simulink model "mdl_r23a"  (R2023a)
settings: Solver=ode1  StartTime=0.0  StopTime=inf  FixedStep=0.1  RelTol=1e-3  EnableMultiTasking=on
values from neighbouring files (symbols this model uses):
  A = 1    [init.m]
  Cn = 30    [init.m]
  Cw = 1.1    [init.m]
  fr = 0.02    [init.m]
  g = 9.81    [init.m]
  i1 = 74/9    (= 8.22222222222)    [init.m]
  i2 = 58/10    (= 5.8)    [init.m]
  Kp = 4000    [init.m]
  m = 455    [init.m]
  m_achse_mitte = Jachse_mitte * i2*i2 / (rR*rR)    (= 1.70347629346)    [init.m]
  m_achse_unten = Jachse_unten / (rR*rR)    (= 0.877732533291)    [init.m]
  m_motor = Jmotor * i1*i1*i2*i2 / (rR*rR)    (= 38.3878032221)    [init.m]
  m_raeder = 4 * Jrad / (rR*rR)    (= 13.5035774353)    [init.m]
  rho = 1.2    [init.m]
  rR = 0.2434    [init.m]
  stop_distance = 10.6182    [init.m]
  Tn = 200    [init.m]
  Un = 48    [init.m]
undefined symbols (not defined in the file or in its folder): f_reibwert, gradient_distance_lookup, gradient_lookup, M_Motor
settings Model: Creator=roustiam  LastModifiedBy=Nico Hörter
settings SolverCC: AlgebraicLoopSolver=TrustRegion
settings DataIOCC: LimitDataPoints=on  SaveFormat=Array  SignalLoggingSaveFormat=ModelDataLogs  ReturnWorkspaceOutputs=off  SignalLoggingName=sigsOut
settings OptimizationCC: BlockReduction=off  BooleanDataType=off  ExpressionDepthLimit=2147483647  InitFltsAndDblsToZero=on  LifeSpan=inf
settings DebuggingCC: SaveWithParameterizedLinksMsg=none  UnderspecifiedInitializationDetection=Classic  MergeDetectMultiDrivingBlocksExec=none  SignalResolutionControl=TryResolveAllWithWarning  MultiTaskDSMMsg=warning  MultiTaskCondExecSysMsg=none  FcnCallInpInsideContextMsg=warning  UnconnectedInputMsg=warning  UnconnectedOutputMsg=warning  UnconnectedLineMsg=warning  StateNameClashWarn=warning  SFUnexpectedBacktrackingDiag=warning  SFNoUnconditionalDefaultTransitionDiag=warning  ArithmeticOperatorsInVariantConditions=warning
settings HardwareCC: ProdBitPerPointer=32  ProdBitPerSizeT=32  ProdBitPerPtrDiffT=32  ProdLargestAtomicFloat=None  ProdIntDivRoundTo=Undefined  ProdEndianess=Unspecified  ProdWordSize=32  ProdHWDeviceType=32-bit Generic  TargetUnknown=on
settings ModelReferenceCC: EnableRefExpFcnMdlSchedulingChecks=on  PropagateSignalLabelsOutOfModel=off
settings SFSimCC: SimUseLocalCustomCode=off  CustomCodeUndefinedFunction=UseInterfaceOnly
settings RTWCC: RTWUseLocalCustomCode=off
settings CodeAppCC: StateflowObjectComments=on
settings GRTTargetCC: TargetFcnLib=ansi_tfl_tmw.mat  TargetLangStandard=C89/C90 (ANSI)  CombineOutputUpdateFcns=off  GRTInterface=on
settings ConfigComp: CovMetricSettings=dw  CovSaveCumulativeToWorkspaceVar=on  CovSaveSingleToWorkspaceVar=on  CovExternalEMLEnable=off

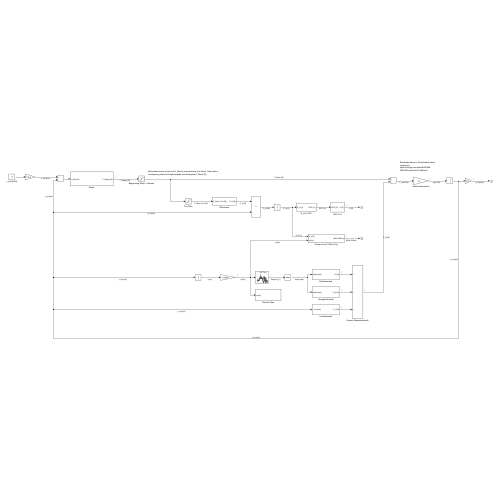
[thumbnail: Simulink's stored preview of the top-level diagram]
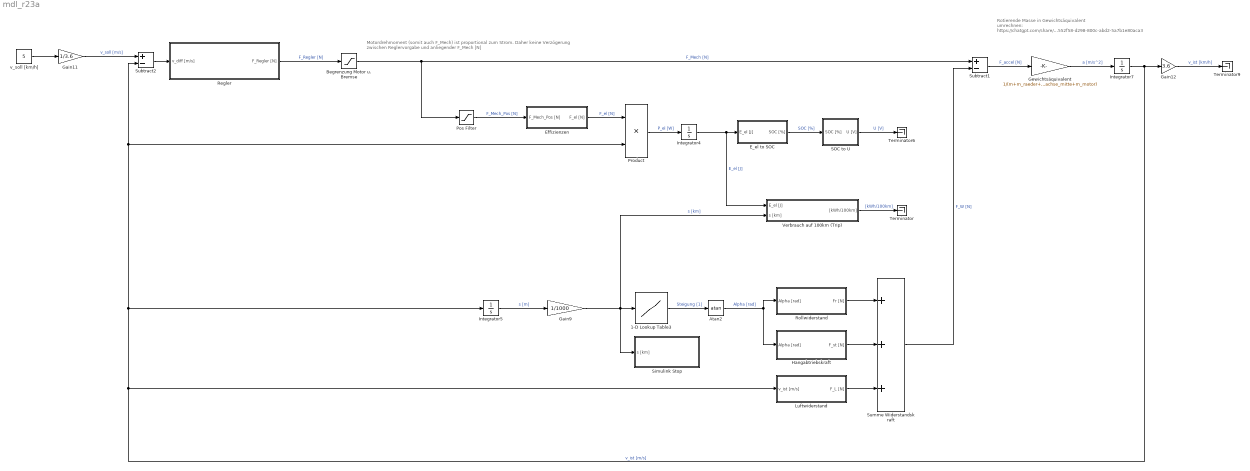
== system mdl_r23a ==
  note: Motordrehmoment (somit auch F_Mech) ist proportional zum Strom. Daher keine Verzögerung zwischen Reglervorgabe und anliegender F_Mech [N]
  note: Rotierende Masse in Gewichtsäquivalent umrechnen:
      | https://chatgpt.com/share/68552f58-d298-800c-abd2-5a7b1e80aca3
  1-D Lookup Table3 : Lookup_n-D  NumberOfTableDimensions=1  BreakpointsForDimension1=gradient_distance_lookup  Table=gradient_lookup  ExtrapMethod=Clip  InternalRulePriority=Speed  RndMeth=Simplest
  Atan2 : Trigonometry  Operator=atan
  Begrenzung Motor u. Bremse : Saturate  UpperLimit=M_Motor*i1*i2/rR  LowerLimit=-f_reibwert*m*g
  E_el to SOC : Subsystem
  Effizienzen : Subsystem
  Gain11 : Gain  Gain=1/3.6
  Gain12 : Gain  Gain=3.6
  Gain9 : Gain  Gain=1/1000
  Gewichtsäquivalent : Gain  Gain=1/(m+m_raeder+m_achse_unten+m_achse_mitte+m_motor)
  Hangabtriebskraft : Subsystem
  Integrator4 : Integrator
  Integrator5 : Integrator
  Integrator7 : Integrator
  Luftwiderstand : Subsystem
  Pos Filter : Saturate  UpperLimit=inf  LowerLimit=0
  Product : Product
  Regler : Subsystem
  Rollwiderstand : Subsystem
  SOC to U : Subsystem
  Simulink Stop : Subsystem
  Subtract1 : Sum  Inputs=+-
  Subtract2 : Sum  Inputs=+-
  Summe Widerstandskraft : Sum  Inputs=+++
  Terminator : Terminator
  Terminator6 : Terminator
  Terminator9 : Terminator
  Verbrauch auf 100km (Trip) : Subsystem
  v_soll [km/h] : Constant  Value=5
  wires:
  Atan2/1 -> Rollwiderstand/1(Alpha [rad]), Hangabtriebskraft/1(Alpha [rad])  "Alpha [rad]"
  1-D Lookup Table3/1 -> Atan2/1  "Steigung [1]"
  Gain9/1 -> Verbrauch auf 100km (Trip)/2(s [km]), Simulink Stop/1(s [km]), 1-D Lookup Table3/1  "s [km]"
  Integrator5/1 -> Gain9/1  "s [m]"
  Rollwiderstand/1(Fr [N]) -> Summe Widerstandskraft/1
  Hangabtriebskraft/1(F_st [N]) -> Summe Widerstandskraft/2
  Luftwiderstand/1(F_L [N]) -> Summe Widerstandskraft/3
  Gewichtsäquivalent/1 -> Integrator7/1  "a [m/s^2]"
  Integrator7/1 -> Product/2, Subtract2/2, Integrator5/1, Luftwiderstand/1(v_ist [m/s]), Gain12/1  "v_ist [m/s]"
  Summe Widerstandskraft/1 -> Subtract1/2  "F_W [N]"
  Regler/1(F_Regler [N]) -> Begrenzung Motor u. Bremse/1  "F_Regler [N]"
  Subtract1/1 -> Gewichtsäquivalent/1  "F_accel [N]"
  v_soll [km/h]/1 -> Gain11/1
  Gain11/1 -> Subtract2/1  "v_soll [m/s]"
  Subtract2/1 -> Regler/1(v_diff [m/s])
  Gain12/1 -> Terminator9/1  "v_ist [km/h]"
  Effizienzen/1(F_el [N]) -> Product/1  "F_el [N]"
  SOC to U/1(U [V]) -> Terminator6/1  "U [V]"
  E_el to SOC/1(SOC [%]) -> SOC to U/1(SOC [%])  "SOC [%]"
  Product/1 -> Integrator4/1  "P_el [W]"
  Integrator4/1 -> E_el to SOC/1(E_el [J]), Verbrauch auf 100km (Trip)/1(E_el [J])  "E_el [J]"
  Pos Filter/1 -> Effizienzen/1(F_Mech_Pos [N])  "F_Mech_Pos [N]"
  Begrenzung Motor u. Bremse/1 -> Subtract1/1, Pos Filter/1  "F_Mech [N]"
  Verbrauch auf 100km (Trip)/1("[kWh/100km]") -> Terminator/1  "[kWh/100km]"

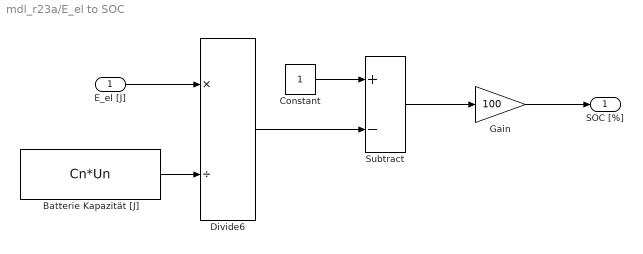
== system mdl_r23a/E_el to SOC ==
  E_el [J] : Inport
  Batterie Kapazität [J] : Constant  Value=Cn*Un
  Constant : Constant
  Divide6 : Product  Inputs=*/
  Gain : Gain  Gain=100
  Subtract : Sum  Inputs=+-
  SOC [%] : Outport
  wires:
  E_el [J]/1 -> Divide6/1
  Batterie Kapazität [J]/1 -> Divide6/2
  Divide6/1 -> Subtract/2
  Constant/1 -> Subtract/1
  Subtract/1 -> Gain/1
  Gain/1 -> SOC [%]/1

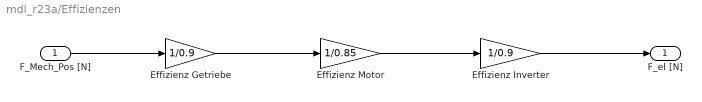
== system mdl_r23a/Effizienzen ==
  F_Mech_Pos [N] : Inport
  Effizienz Getriebe : Gain  Gain=1/0.9
  Effizienz Inverter : Gain  Gain=1/0.9
  Effizienz Motor : Gain  Gain=1/0.85
  F_el [N] : Outport
  wires:
  Effizienz Getriebe/1 -> Effizienz Motor/1
  Effizienz Motor/1 -> Effizienz Inverter/1
  Effizienz Inverter/1 -> F_el [N]/1
  F_Mech_Pos [N]/1 -> Effizienz Getriebe/1

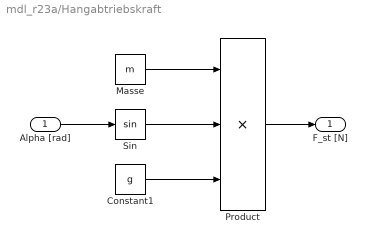
== system mdl_r23a/Hangabtriebskraft ==
  Alpha [rad] : Inport
  Constant1 : Constant  Value=g
  Masse : Constant  Value=m
  Product : Product  Inputs=3
  Sin : Trigonometry
  F_st [N] : Outport
  wires:
  Product/1 -> F_st [N]/1
  Masse/1 -> Product/1
  Sin/1 -> Product/2
  Alpha [rad]/1 -> Sin/1
  Constant1/1 -> Product/3

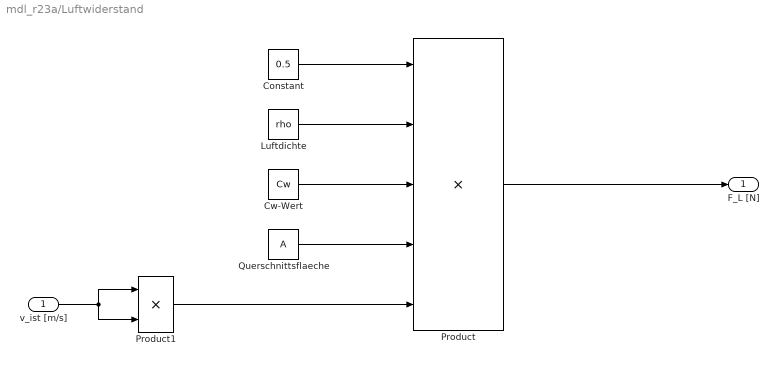
== system mdl_r23a/Luftwiderstand ==
  v_ist [m/s] : Inport
  Constant : Constant  Value=0.5
  Cw-Wert : Constant  Value=Cw
  Luftdichte : Constant  Value=rho
  Product : Product  Inputs=5
  Product1 : Product
  Querschnittsflaeche : Constant  Value=A
  F_L [N] : Outport
  wires:
  Querschnittsflaeche/1 -> Product/4
  Cw-Wert/1 -> Product/3
  Luftdichte/1 -> Product/2
  Constant/1 -> Product/1
  Product1/1 -> Product/5
  v_ist [m/s]/1 -> Product1/1, Product1/2
  Product/1 -> F_L [N]/1

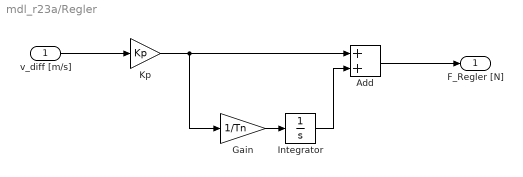
== system mdl_r23a/Regler ==
  v_diff [m/s] : Inport
  Add : Sum
  Gain : Gain  Gain=1/Tn
  Integrator : Integrator
  Kp : Gain  Gain=Kp
  F_Regler [N] : Outport
  wires:
  v_diff [m/s]/1 -> Kp/1
  Add/1 -> F_Regler [N]/1
  Kp/1 -> Add/1, Gain/1
  Gain/1 -> Integrator/1
  Integrator/1 -> Add/2

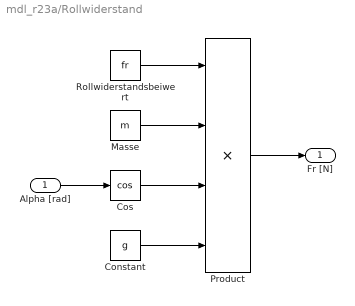
== system mdl_r23a/Rollwiderstand ==
  Alpha [rad] : Inport
  Constant : Constant  Value=g
  Cos : Trigonometry  Operator=cos
  Masse : Constant  Value=m
  Product : Product  Inputs=4
  Rollwiderstandsbeiwert : Constant  Value=fr
  Fr [N] : Outport
  wires:
  Alpha [rad]/1 -> Cos/1
  Product/1 -> Fr [N]/1
  Constant/1 -> Product/4
  Cos/1 -> Product/3
  Masse/1 -> Product/2
  Rollwiderstandsbeiwert/1 -> Product/1

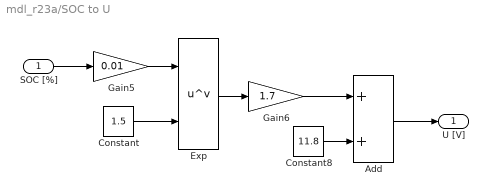
== system mdl_r23a/SOC to U ==
  SOC [%] : Inport
  Add : Sum
  Constant : Constant  Value=1.5
  Constant8 : Constant  Value=11.8
  Exp : Math  Operator=pow
  Gain5 : Gain  Gain=0.01
  Gain6 : Gain  Gain=1.7
  U [V] : Outport
  wires:
  Constant/1 -> Exp/2
  Gain6/1 -> Add/1
  Exp/1 -> Gain6/1
  Gain5/1 -> Exp/1
  Constant8/1 -> Add/2
  SOC [%]/1 -> Gain5/1
  Add/1 -> U [V]/1

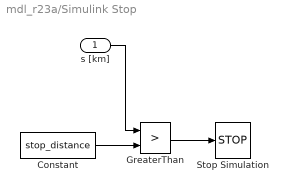
== system mdl_r23a/Simulink Stop ==
  s [km] : Inport
  Constant : Constant  Value=stop_distance
  GreaterThan : RelationalOperator  Operator=>  OutDataTypeStr=boolean  RndMeth=Simplest  InputSameDT=off
  Stop Simulation : Stop
  wires:
  s [km]/1 -> GreaterThan/1
  GreaterThan/1 -> Stop Simulation/1
  Constant/1 -> GreaterThan/2

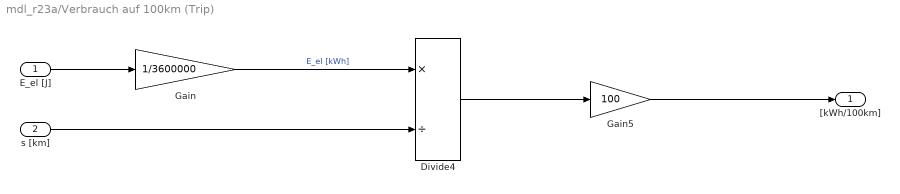
== system mdl_r23a/Verbrauch auf 100km (Trip) ==
  E_el [J] : Inport
  s [km] : Inport  Port=2
  Divide4 : Product  Inputs=*/
  Gain : Gain  Gain=1/3600000
  Gain5 : Gain  Gain=100
  "[kWh/100km]" : Outport
  wires:
  Divide4/1 -> Gain5/1
  Gain/1 -> Divide4/1  "E_el [kWh]"
  E_el [J]/1 -> Gain/1
  Gain5/1 -> "[kWh/100km]"/1
  s [km]/1 -> Divide4/2
